simulink model "autopilota_v_22_last"  (R2020b)
(part 9 of 12)

      0, 0, 0,                                                                                                                                                                                                                                                                                                                                                                                                                                                                                                                                                                                                                                                                                                                                                                                                                                0,                                                                                                                                                                                                                                                                                                                                                                                                                                                                                                                                                                                                                                                                                                                                                                                                                                0, 0,                                                                                                                                                                                                                                                                                                                                                                                                                                                                                                                                                                                                                                                                                                                                                                                                                                                                                                                                                                                                                                                                                                                                                                                                                                                                                                                                                                                                                                                                                                                                                       0,                                                                                                                                                                                                                                                                                                                                                                                                                                                                                                                                                                                                                                                                                                                                                                                                                                                                                                                                                                                                                                                                                                                                                                                                                                                                                                                                                                                                                                                                                                                                                    0,                                                                                                                                                                                                                                                                                                                                                                                                                                                                                                                                                                                                                                                                                                                                                                                                                                                                                                                                                                                                                                                                                                                                                                                                                                                                                                                                                                                                                                                                                                                                                                                                                                           0,                                                0,                                                0,                   0,                                                                                                                                                                                                                                                                                                                                                                                                                                                                                                                                                                                                                                                                                                                                                                                                                                                                                                                                                                                                                                                                                                                                                                                                                                                                                                                                                                                                                                                                                               0,                                                                                                                                                                                                                                                                                                                                                                                                                                                                                                                                                                                                                                                                                                                                                                                                                                                                                                                                                                                                                                                                                                                                                                                                                                                                                                                                                                                                                                  0,                                                                                                                                                                                                                                                                                                                                                                                                                                                                                                                                                                                                                                                                                                                                                                                                                                                                                                                                                                                                                                                                                                                                                                                                                                                                                                                                                                                                                                  1, 0, 0, 0, 0, 0, 1;...
      0, 0, 0,                                                                                                                                                                                                                                                                                                                                                                                                                                                                                                                                                                                                                                                                                                                                                                                                                                0,                                                                                                                                                                                                                                                                                                                                                                                                                                                                                                                                                                                                                                                                                                                                                                                                                                0, 0,                                                                                                                                                                                                                                                                                                                                                                                                                                                                                                                                                                                                                                                                                                                                                                                                                                                                                                                                                                                                                                                                                                                                                                                                                                                                                                                                                                                                                                                                                                                                                       0,                                                                                                                                                                                                                                                                                                                                                                                                                                                                                                                                                                                                                                                                                                                                                                                                                                                                                                                                                                                                                                                                                                                                                                                                                                                                                                                                                                                                                                                                        - cos(theta)*(ad - 981/100) - an*cos(psi)*sin(theta) - ae*sin(psi)*sin(theta),                                                                                                                                                                                                                                                                                                                                                                                                                                                                                                                                                                                                                                                                                                                                                                                                                                                                                                                                                                                                                                                                                                                                                                                                                                                                                                                                                                                                                                                                                                                                                                                             ae*cos(psi)*cos(theta) - an*cos(theta)*sin(psi),                              cos(psi)*cos(theta),                              cos(theta)*sin(psi),         -sin(theta),                                                                                                                                                                                                                                                                                                                                                                                                                                                                                                                                                                                                                                                                                                                                                                                                                                                                                                                                                                                                                                                                                                                                                                                                                                                                                                                                                                                                                                                                               q*ryIMU + r*rzIMU,                                                                                                                                                                                                                                                                                                                                                                                                                                                                                                                                                                                                                                                                                                                                                                                                                                                                                                                                                                                                                                                                                                                                                                                                                                                                                                                                                                                                                p*ryIMU - 2*q*rxIMU,                                                                                                                                                                                                                                                                                                                                                                                                                                                                                                                                                                                                                                                                                                                                                                                                                                                                                                                                                                                                                                                                                                                                                                                                                                                                                                                                                                                                                p*rzIMU - 2*r*rxIMU, 1, 0, 0, 0, 0, 0;...
      0, 0, 0,                                                                                                                                                                                                                                                                                                                                                                                                                                                                                                                                                                                                                                                                                                                                                                                                                                0,                                                                                                                                                                                                                                                                                                                                                                                                                                                                                                                                                                                                                                                                                                                                                                                                                                0, 0,                                                                                                                                                                                                                                                                                                                                                                                                                                                                                                                                                                                                                                                                                                                                                                                                                                                                                                                                                                                                                                                                                                                                                                                                                                                                                                                                                                                                      an*(sin(phi)*sin(psi) + cos(phi)*cos(psi)*sin(theta)) - ae*(cos(psi)*sin(phi) - cos(phi)*sin(psi)*sin(theta)) + cos(phi)*cos(theta)*(ad - 981/100),                                                                                                                                                                                                                                                                                                                                                                                                                                                                                                                                                                                                                                                                                                                                                                                                                                                                                                                                                                                                                                                                                                                                                                                                                                                                                                                                                                                                                                               an*cos(psi)*cos(theta)*sin(phi) - sin(phi)*sin(theta)*(ad - 981/100) + ae*cos(theta)*sin(phi)*sin(psi),                                                                                                                                                                                                                                                                                                                                                                                                                                                                                                                                                                                                                                                                                                                                                                                                                                                                                                                                                                                                                                                                                                                                                                                                                                                                                                                                                                                                                                                                                                                             - ae*(cos(phi)*sin(psi) - cos(psi)*sin(phi)*sin(theta)) - an*(cos(phi)*cos(psi) + sin(phi)*sin(psi)*sin(theta)), cos(psi)*sin(phi)*sin(theta) - cos(phi)*sin(psi), cos(phi)*cos(psi) + sin(phi)*sin(psi)*sin(theta), cos(theta)*sin(phi),                                                                                                                                                                                                                                                                                                                                                                                                                                                                                                                                                                                                                                                                                                                                                                                                                                                                                                                                                                                                                                                                                                                                                                                                                                                                                                                                                                                                                                                                             q*rxIMU - 2*p*ryIMU,                                                                                                                                                                                                                                                                                                                                                                                                                                                                                                                                                                                                                                                                                                                                                                                                                                                                                                                                                                                                                                                                                                                                                                                                                                                                                                                                                                                                                  p*rxIMU + r*rzIMU,                                                                                                                                                                                                                                                                                                                                                                                                                                                                                                                                                                                                                                                                                                                                                                                                                                                                                                                                                                                                                                                                                                                                                                                                                                                                                                                                                                                                                q*rzIMU - 2*r*ryIMU, 0, 1, 0, 0, 0, 0;...
      0, 0, 0,                                                                                                                                                                                                                                                                                                                                                                                                                                                                                                                                                                                                                                                                                                                                                                                                                                0,                                                                                                                                                                                                                                                                                                                                                                                                                                                                                                                                                                                                                                                                                                                                                                                                                                0, 0,                                                                                                                                                                                                                                                                                                                                                                                                                                                                                                                                                                                                                                                                                                                                                                                                                                                                                                                                                                                                                                                                                                                                                                                                                                                                                                                                                                                                      an*(cos(phi)*sin(psi) - cos(psi)*sin(phi)*sin(theta)) - ae*(cos(phi)*cos(psi) + sin(phi)*sin(psi)*sin(theta)) - cos(theta)*sin(phi)*(ad - 981/100),                                                                                                                                                                                                                                                                                                                                                                                                                                                                                                                                                                                                                                                                                                                                                                                                                                                                                                                                                                                                                                                                                                                                                                                                                                                                                                                                                                                                                                               an*cos(phi)*cos(psi)*cos(theta) - cos(phi)*sin(theta)*(ad - 981/100) + ae*cos(phi)*cos(theta)*sin(psi),                                                                                                                                                                                                                                                                                                                                                                                                                                                                                                                                                                                                                                                                                                                                                                                                                                                                                                                                                                                                                                                                                                                                                                                                                                                                                                                                                                                                                                                                                                                               ae*(sin(phi)*sin(psi) + cos(phi)*cos(psi)*sin(theta)) + an*(cos(psi)*sin(phi) - cos(phi)*sin(psi)*sin(theta)), sin(phi)*sin(psi) + cos(phi)*cos(psi)*sin(theta), cos(phi)*sin(psi)*sin(theta) - cos(psi)*sin(phi), cos(phi)*cos(theta),                                                                                                                                                                                                                                                                                                                                                                                                                                                                                                                                                                                                                                                                                                                                                                                                                                                                                                                                                                                                                                                                                                                                                                                                                                                                                                                                                                                                                                                                             r*rxIMU - 2*p*rzIMU,                                                                                                                                                                                                                                                                                                                                                                                                                                                                                                                                                                                                                                                                                                                                                                                                                                                                                                                                                                                                                                                                                                                                                                                                                                                                                                                                                                                                                r*ryIMU - 2*q*rzIMU,                                                                                                                                                                                                                                                                                                                                                                                                                                                                                                                                                                                                                                                                                                                                                                                                                                                                                                                                                                                                                                                                                                                                                                                                                                                                                                                                                                                                                  p*rxIMU + q*ryIMU, 0, 0, 1, 0, 0, 0];


%% Measurement noise covariance %%
%%%%%%%%%%%%%%%%%%%%%%%%%%%%%%%%%%

R = [ 3.5e-11;...%Lat
      3.5e-11;...%Long
      0.8241;...%h(press)
      1.7e-5;...%v
      1.7e-3;...%psi(GPS)
      1.7e-4;...%vd
      6e-05	;...%phi
      6e-05;...%theta
      6e-08;...%psi
      3.18e-05;...%p
      2.42e-05;...%q
      4.18e-05;...%r
      4.13e-05;...%ax
      4.13e-05;...%ay
      8.29e-05];  %az 
  
%%%%%%%%%%%%%%%%%%%%%%%%  
%% Measurement update %%
%%%%%%%%%%%%%%%%%%%%%%%%

% Estimation
S = H * p_prd' * H';

if clock_GPS==1 && clock_MTi==1
    
    for i = 1:15
        
        S(i,i) = S(i,i) + R(i);
        
    end
		 
elseif clock_GPS==0 && clock_MTi==0 
    
    for i = 1:15
        
        if i==3
            
            S(i,i) = S(i,i) + R(i);
        
        else
            
            S(i,i) = S(i,i) + infinito;
            
        end
        
    end

else
    
    for i = 1:15
        
        if i==3 || i>=7
            
			S(i,i) = S(i,i) + R(i);
        
		else
            
			S(i,i) = S(i,i) + infinito;
        
        end
        
    end
		 
end

B = H * p_prd';
klm_gain = (S \ B)';

% Estimated state and covariance
%---------Inizio modifiche rispetto all'originale per correggere il salto
%dell'heading quando  si va verso 180

errore_prd = (Z - Y_prd);

    if ((-pi <= Z(5) && Z(5) < -pi/2) && (pi >= Y_prd(5) && Y_prd(5) > pi/2) && Z(5)*Y_prd(5) < 0)
        errore_prd(5) = mod(Z(5) - Y_prd(5),2*pi);
    elseif ((pi >= Z(5) && Z(5) > pi/2) && (-pi <= Y_prd(5) && Y_prd(5) < -pi/2) && Z(5)*Y_prd(5) < 0)
        errore_prd(5) = (Z(5) - Y_prd(5)) - 2*pi;
    end
    
    if ((-pi <= Z(9) && Z(9) < -pi/2) && (pi >= Y_prd(9) && Y_prd(9) > pi/2) && Z(9)*Y_prd(9) < 0)
        errore_prd(9) = mod(Z(9) - Y_prd(9),2*pi);
    elseif ((pi >= Z(9) && Z(9) > pi/2) && (-pi <= Y_prd(9) && Y_prd(9) < -pi/2) && Z(9)*Y_prd(9) < 0)
        errore_prd(9) = (Z(9) - Y_prd(9)) - 2*pi;
    end
    
x_est = x_prd + klm_gain * (errore_prd);
p_est = p_prd - klm_gain * H * p_prd;

%fine delle correzzioni------------%
%%%%%%%%%%%%%%%%%%%%%%%%
%% Linearize dynamics %%
%%%%%%%%%%%%%%%%%%%%%%%%

lat = x_est(1); long = x_est(2); h = x_est(3); vn = x_est(4); ve = x_est(5); vd = x_est(6); phi  = x_est(7); theta = x_est(8); psi = x_est(9);

an  = x_est(10); ae = x_est(11); ad = x_est(12); p = x_est(13); q = x_est(14); r = x_est(15); baccx = x_est(16); baccy = x_est(17); baccz = x_est(18); bp = x_est(19); bq = x_est(20); br = x_est(21);


F = [                                           1, 0,            -(dt*vn)/(h + 6378137)^2, dt/(h + 6378137),                           0,   0,                                           0,                                                      0, 0,  0,  0,  0,  0,                        0,                        0, 0, 0, 0, 0, 0, 0;...
      (dt*ve*sin(lat))/(cos(lat)^2*(h + 6378137)), 1, -(dt*ve)/(cos(lat)*(h + 6378137)^2),                0, dt/(cos(lat)*(h + 6378137)),   0,                                           0,                                                      0, 0,  0,  0,  0,  0,                        0,                        0, 0, 0, 0, 0, 0, 0;...
                                                0, 0,                                   1,                0,                           0, -dt,                                           0,                                                      0, 0,  0,  0,  0,  0,                        0,                        0, 0, 0, 0, 0, 0, 0;...
                                                0, 0,                                   0,                1,                           0,   0,                                           0,                                                      0, 0, dt,  0,  0,  0,                        0,                        0, 0, 0, 0, 0, 0, 0;...
                                                0, 0,                                   0,                0,                           1,   0,                                           0,                                                      0, 0,  0, dt,  0,  0,                        0,                        0, 0, 0, 0, 0, 0, 0;...
                                                0, 0,                                   0,                0,                           0,   1,                                           0,                                                      0, 0,  0,  0, dt,  0,                        0,                        0, 0, 0, 0, 0, 0, 0;...
                                                0, 0,                                   0,                0,                           0,   0, dt*tan(theta)*(q*cos(phi) - r*sin(phi)) + 1,        dt*(tan(theta)^2 + 1)*(r*cos(phi) + q*sin(phi)), 0,  0,  0,  0, dt,   dt*sin(phi)*tan(theta),   dt*cos(phi)*tan(theta), 0, 0, 0, 0, 0, 0;...
                                                0, 0,                                   0,                0,                           0,   0,               -dt*(r*cos(phi) + q*sin(phi)),                                                      1, 0,  0,  0,  0,  0,              dt*cos(phi),             -dt*sin(phi), 0, 0, 0, 0, 0, 0;...
                                                0, 0,                                   0,                0,                           0,   0,   (dt*(q*cos(phi) - r*sin(phi)))/cos(theta), (dt*sin(theta)*(r*cos(phi) + q*sin(phi)))/cos(theta)^2, 1,  0,  0,  0,  0, (dt*sin(phi))/cos(theta), (dt*cos(phi))/cos(theta), 0, 0, 0, 0, 0, 0;...
                                                0, 0,                                   0,                0,                           0,   0,                                           0,                                                      0, 0,  1,  0,  0,  0,                        0,                        0, 0, 0, 0, 0, 0, 0;...
                                                0, 0,                                   0,                0,                           0,   0,                                           0,                                                      0, 0,  0,  1,  0,  0,                        0,                        0, 0, 0, 0, 0, 0, 0;...
                                                0, 0,                                   0,                0,                           0,   0,                                           0,                                                      0, 0,  0,  0,  1,  0,                        0,                        0, 0, 0, 0, 0, 0, 0;...
                                                0, 0,                                   0,                0,                           0,   0,                                           0,                                                      0, 0,  0,  0,  0,  1,                        0,                        0, 0, 0, 0, 0, 0, 0;...
                                                0, 0,                                   0,                0,                           0,   0,                                           0,                                                      0, 0,  0,  0,  0,  0,                        1,                        0, 0, 0, 0, 0, 0, 0;...
                                                0, 0,                                   0,                0,                           0,   0,                                           0,                                                      0, 0,  0,  0,  0,  0,                        0,                        1, 0, 0, 0, 0, 0, 0;...
                                                0, 0,                                   0,                0,                           0,   0,                                           0,                                                      0, 0,  0,  0,  0,  0,                        0,                        0, 1, 0, 0, 0, 0, 0;...
                                                0, 0,                                   0,                0,                           0,   0,                                           0,                                                      0, 0,  0,  0,  0,  0,                        0,                        0, 0, 1, 0, 0, 0, 0;...
                                                0, 0,                                   0,                0,                           0,   0,                                           0,                                                      0, 0,  0,  0,  0,  0,                        0,                        0, 0, 0, 1, 0, 0, 0;...
                                                0, 0,                                   0,                0,                           0,   0,                                           0,                                                      0, 0,  0,  0,  0,  0,                        0,                        0, 0, 0, 0, 1, 0, 0;...
                                                0, 0,                                   0,                0,                           0,   0,                                           0,                                                      0, 0,  0,  0,  0,  0,                        0,                        0, 0, 0, 0, 0, 1, 0;...
                                                0, 0,                                   0,                0,                           0,   0,                                           0,                                                      0, 0,  0,  0,  0,  0,                        0,                        0, 0, 0, 0, 0, 0, 1];

%%%%%%%%%%%%%%%%%                                            
%% Time update %%
%%%%%%%%%%%%%%%%%

% Predicted (nonlinear) state

x_prd(1) = lat + ( vn/(a+h) )*dt;
x_prd(2) = long + ( ve/((a+h)*cos(lat)) )*dt;
x_prd(3) = h -vd*dt;
x_prd(4) = vn + an*dt;
x_prd(5) = ve + ae*dt;
x_prd(6) = vd + ad*dt;
x_prd(7)  = phi + ( ( q*sin(phi)+r*cos(phi) )*tan(theta)+p )*dt;
x_prd(8)  = theta + ( q*cos(phi)-r*sin(phi) )*dt;
x_prd(9)  = mod( (psi + ( ( q*sin(phi)+r*cos(phi) )*(1/cos(theta)) )*dt)+pi,2*pi )-pi;
x_prd(10)  = an;
x_prd(11)  = ae;
x_prd(12)  = ad;
x_prd(13)  = p;
x_prd(14)  = q;
x_prd(15)  = r;
x_prd(16) = baccx;
x_prd(17) = baccy;
x_prd(18) = baccz;
x_prd(19) = bp;
x_prd(20) = bq;
x_prd(21) = br;

% Predicted covariance



p_prd = F * p_est * F';

for k = 1:21
    
    p_prd(k,k) = p_prd(k,k) + Q(k);
    
end

%%%%%%%%%%
%% Exit %%
%%%%%%%%%%  

Lat_K = x_est(1);
Long_K = x_est(2);
h_K = x_est(3);
v_K = sqrt( ((x_est(4))^2)+((x_est(5))^2));
vd_K = x_est(6);
phi_K = x_est(7);
theta_K = x_est(8);
psi_K = atan2(x_est(5),x_est(4));
p_K = x_est(13);
q_K = x_est(14);
r_K = x_est(15);
errore_5 = errore_prd(5);
errore_9 = errore_prd(9);
imbardata = x_est(9);
